simulink model "prbs_model"  (R2022a)
settings: Solver=ode4  StartTime=0.0  StopTime=10  FixedStep=0.0005  RelTol=1e-3
settings Model: Creator=randolf  LastModifiedBy=randolf

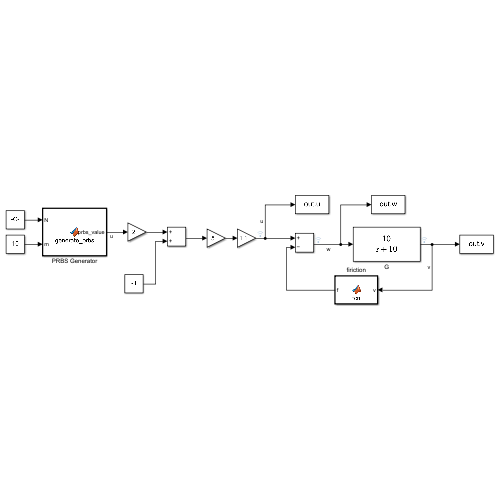
[thumbnail: Simulink's stored preview of the top-level diagram]
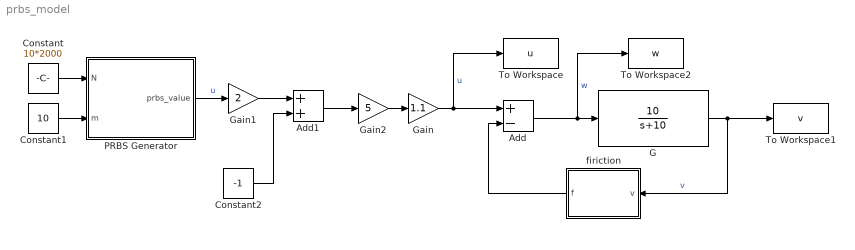
== system prbs_model ==
  Add : Sum  Inputs=+-
  Add1 : Sum
  Constant : Constant  Value=10*2000
  Constant1 : Constant  Value=10
  Constant2 : Constant  Value=-1
  G : TransferFcn  Numerator=[10]  Denominator=[1 10]
  Gain : Gain  Gain=1.1
  Gain1 : Gain  Gain=2
  Gain2 : Gain  Gain=5
  PRBS Generator : MATLAB Function  TreatAsAtomicUnit=on
  To Workspace : ToWorkspace  VariableName=u  SaveFormat=Timeseries  SampleTime=-1
  To Workspace1 : ToWorkspace  VariableName=v  SaveFormat=Timeseries  SampleTime=-1
  To Workspace2 : ToWorkspace  VariableName=w  SaveFormat=Timeseries  SampleTime=-1
  firiction : MATLAB Function  TreatAsAtomicUnit=on
  wires:
  G/1 -> To Workspace1/1, firiction/1(v)  "v"
  Add/1 -> To Workspace2/1, G/1  "w"
  firiction/1(f) -> Add/2
  Gain/1 -> To Workspace/1, Add/1  "u"
  Constant/1 -> PRBS Generator/1(N)
  Constant1/1 -> PRBS Generator/2(m)
  PRBS Generator/1(prbs_value) -> Gain1/1  "u"
  Constant2/1 -> Add1/2
  Gain1/1 -> Add1/1
  Add1/1 -> Gain2/1
  Gain2/1 -> Gain/1

== matlab function prbs_model/firiction ==
  data: v input; f output
function f = fcn(v)
    if (v>0)
        f = 0.5;
    else
        f = -0.4;
    end
end

== matlab function prbs_model/PRBS Generator ==
  data: N input; prbs_value output; m input
function prbs_value = generate_prbs(N, m)
% 生成 PRBS 信号
% N - 序列长度
% m - 移位寄存器的阶数

persistent shift_register prbs_signal index

if isempty(shift_register)
    % 初始化移位寄存器
    shift_register = ones(1, m);
    % 初始化 PRBS 信号
    prbs_signal = zeros(1, N);
    index = 1;
    
    % 生成完整的 PRBS 信号
    for i = 1:N
        % 计算反馈位
        feedback = xor(shift_register(m), shift_register(m - 1));

        % 更新 PRBS 信号
        prbs_signal(i) = shift_register(m);

        % 更新移位寄存器
        shift_register = [feedback, shift_register(1:m - 1)];
    end
end

% 输出当前 PRBS 信号值
prbs_value = prbs_signal(index);

% 更新索引
index = index + 1;
if index > N
    index = 1; % 循环使用 PRBS 信号
end
end
